simulink model "WashMachine_2018a"  (R2020a)
settings: Solver=VariableStepAuto  StartTime=0.0  StopTime=10.0  RelTol=1e-3
settings Model: Creator=apple  LastModifiedBy=bzhan
settings DebuggingCC: ArithmeticOperatorsInVariantConditions=warning
settings SFSimCC: CustomCodeUndefinedFunction=UseInterfaceOnly

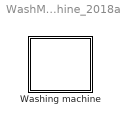
== system WashMachine_2018a ==
  Washing machine : Stateflow chart  TreatAsAtomicUnit=on

== stateflow chart WashMachine_2018a/Washing machine ==
  state On
    on E:fprintf("Washing Completed!");
    (history)
    state AddWater
      du:time = time + 1;
      en:fprintf("Add water")
    state Washing
      du:time = time + 1;
      en:fprintf("Washing")
    AddWater -> Washing : [time>=5]/{time=0;}
    Washing -> AddWater : [time>=10]/{time=0;}
  state Off
    state Ready
      en:fprintf("Init");
      remain = 45;
    state Sleep
      en:time = 0;
      finish = 0;
    state Pending
      en:fprintf("pending")
    (default) -> Sleep
    Sleep -> Ready : START
    Pending -> Sleep [order 1] : STOP
  (default) -> Off
  Ready -> AddWater : SWITCH
  On -> Off [order 1] : STOP
  On -> Off [order 3] : after(remain,sec)[finish == 0]{finish = 1;send(E);}
  Pending -> On [order 2] : SWITCH
  On -> Pending [order 2] : SWITCH{remain=remain-temporalCount(sec)}
  data: remain local =45; finish local; time local
  events: E local FUNCTION_CALL_EVENT; SWITCH local RISING_EDGE_EVENT; START local FUNCTION_CALL_EVENT; STOP local FUNCTION_CALL_EVENT
